simulink model "tsep"  (R2020a)
settings: Solver=ode15s  StartTime=0.0  StopTime=3600  RelTol=1e-4
undefined symbols (not defined in the file or in its folder): qci, qwi
settings Model: Creator=sho  LastModifiedBy=sho

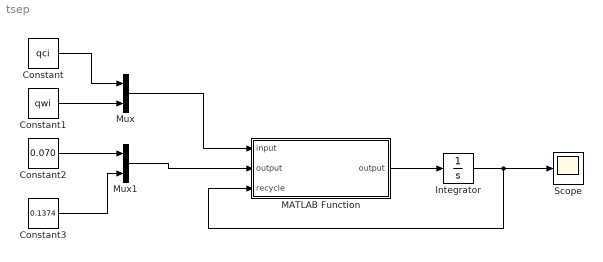
== system tsep ==
  Constant : Constant  Value=qci
  Constant1 : Constant  Value=qwi
  Constant2 : Constant  Value=0.070
  Constant3 : Constant  Value=0.1374
  Integrator : Integrator  InitialCondition=[0.01,0.01]
  MATLAB Function : MATLAB Function  TreatAsAtomicUnit=on
  Mux : Mux  Inputs=2
  Mux1 : Mux  Inputs=2
  Scope : Scope
  wires:
  Mux/1 -> MATLAB Function/1(input)
  Mux1/1 -> MATLAB Function/2("output ")
  Constant/1 -> Mux/1
  Constant1/1 -> Mux/2
  Constant2/1 -> Mux1/1
  Constant3/1 -> Mux1/2
  MATLAB Function/1(output) -> Integrator/1
  Integrator/1 -> MATLAB Function/3(recycle), Scope/1

== matlab function tsep/MATLAB Function ==
  data: input input; output output; output input; recycle input; const parameter
function output = tseptmodel(input,output,recycle,const)

% Inputs
qci = input(1);         % Inflow of oil (m3/s)
qwi = input(2);         % Inflow of water (m3/s)
qca = output(1);        % Outflow of oil (m3/s)
qwo = output(2);        % Outflow of oil (m3/s)

% Geometric parameters
La = const(1);
D = const(2);
Lb = const(3);
hs = const(4);

% Recycle signals
ha = recycle(1);
hw = recycle(2);

% Oil water separator system fluid level ha
dha = (qci + qwi-qca-qwo)/hemihead(ha,La,D);

% Water bed subsystem fluid level hw
dhw = (qwi-qwo)/hemihead(hw,Lb,D);

output = [dha; dhw];
